simulink model "modelo_f"  (R2024b)
settings: Solver=ode15s  StartTime=0.0  StopTime=inf  FixedStep=T_s  RelTol=1e-3
InitFcn:
  | clc
  | clear
  | close all
  | clear all
  | clear mex
  | parametros
  | gain_CL
  | calculo_observador_carro
  | calculo_observador_izaje
values from neighbouring files (symbols this model uses):
  b_cx = 1e6    (= 1000000)    [parametros.m]
  b_cy = 1e7    (= 10000000)    [parametros.m]
  b_hb = 1e8    (= 100000000)    [parametros.m]
  b_hd = 8    [parametros.m]
  b_hm = 18    [parametros.m]
  b_t = 90    [parametros.m]
  b_tb = 5e6    (= 5000000)    [parametros.m]
  b_td = 1.8    [parametros.m]
  b_tm = 6    [parametros.m]
  b_tw = 3e3    (= 3000)    [parametros.m]
  b_wu = 150    [parametros.m]
  container_pillars = container_pillars(randperm(19))    [parametros.m]
  dx_grid_lidar = 0.01    [parametros.m]
  escenario = 1    [parametros.m]
  g = 9.80665    [parametros.m]
  H_c = 2.59    [parametros.m]
  H_truck = 1    [parametros.m]
  i_h = 22    [parametros.m]
  i_t = 30    [parametros.m]
  J_hd_hEb = 3800    [parametros.m]
  J_hm_hb = 30    [parametros.m]
  J_td = 1200    [parametros.m]
  J_tm_tb = 7    [parametros.m]
  K_cy = 1.8e9    (= 1800000000)    [parametros.m]
  K_tw = 4.8e5    (= 480000)    [parametros.m]
  k_wu = 2.36e8    (= 236000000)    [parametros.m]
  l_h0 = (Y_t0-y_l0)    (= 38)    [parametros.m]
  l_h_max = Y_t0-y_h_min    (= 65)    [parametros.m]
  l_h_maxE = l_h_max+0.5    (= 65.5)    [parametros.m]
  l_h_min = Y_t0-y_h_max    (= 5)    [parametros.m]
  l_h_minE = l_h_min-0.5    (= 4.5)    [parametros.m]
  Lt = place(At', Ct', polos_deseados)'    [calculo_observador_carro.m]
  M_cmax = 50000    [parametros.m]
  M_cmin = 2000    [parametros.m]
  M_s = 15000    [parametros.m]
  M_t = 30000    [parametros.m]
  r_hd = 0.75    [parametros.m]
  r_td = 0.50    (= 0.5)    [parametros.m]
  T_hbMax = 5e4    (= 50000)    [parametros.m]
  T_hEbMax = 1.1e6    (= 1100000)    [parametros.m]
  T_hmMax = 2e4    (= 20000)    [parametros.m]
  T_s = 0.001    [parametros.m]
  T_s0 = 0.001    [parametros.m]
  T_s1 = 0.020    (= 0.02)    [parametros.m]
  T_s2 = 0.020    (= 0.02)    [parametros.m]
  T_tbMax = 5e3    (= 5000)    [parametros.m]
  T_tmMax = 4e3    (= 4000)    [parametros.m]
  tau_tm = 1e-3    (= 0.001)    [parametros.m]
  theta_hm0 = -l_h0*i_h*2/r_hd    (= -2229.33333333)    [parametros.m]
  theta_tm0 = (x_t0)*i_t/r_td    (= -900)    [parametros.m]
  trucks0 = [0, 0, 0, 0, 0]    [parametros.m]
  v_h_max_load = 1.5    [parametros.m]
  v_h_max_noload = 3    [parametros.m]
  v_lx0 = 0    [parametros.m]
  v_ly0 = 0    [parametros.m]
  v_t0 = 0    [parametros.m]
  v_t_max = 4    [parametros.m]
  W_c = ctrb(A, B_c(:,1))    [CyO_carro.m]    (also in CyO_izaje.m; parametros.m = 2.44)
  w_hm0 = 0    [parametros.m]
  w_hm_min_BRK = 0.005    [parametros.m]
  w_hm_rated = v_h_max_load*2*i_h/r_hd    (= 88)    [parametros.m]
  w_tm0 = (v_t0)*i_t/r_td    (= 0)    [parametros.m]
  w_tm_min_BRK = 0.005    [parametros.m]
  x_c0_left = -35    [parametros.m]
  x_c0_right = 55    [parametros.m]
  x_containers_left_lim = 1.5    [parametros.m]
  x_containers_right_lim = 48.5    [parametros.m]
  x_l0 = x_t0    (= -15)    [parametros.m]
  x_lidar_offset = 3.0    (= 3)    [parametros.m]
  x_t0 = -15    [parametros.m]
  x_t_max = 50    [parametros.m]
  x_t_maxE = x_t_max+0.5    (= 50.5)    [parametros.m]
  x_t_min = -30    [parametros.m]
  x_t_minE = x_t_min-0.5    (= -30.5)    [parametros.m]
  y_h_min = -20    [parametros.m]
  y_l0 = 7    [parametros.m]
  Y_sb = 5.0    (= 5)    [parametros.m]
  Y_t0 = 45    [parametros.m]
undefined symbols (not defined in the file or in its folder): Lh, parametros
libraries: dspnetwork x2, dspsigops x1, simulink x1
(part 4 of 4)

== stateflow chart modelo_f/Chart ==
  state Nivel_1
    state Heartbeat_Generator [parallel]
      settings: executionOrder=1
      state Heartbeat_High
        entry:
        heartbeat = true;
      state Heartbeat_Low
        entry:
        heartbeat = false;
      (default) -> Heartbeat_High
      Heartbeat_Low -> Heartbeat_High : after(200, msec)
      Heartbeat_High -> Heartbeat_Low : after(200, msec)
    state Supervisory_Control [parallel]
      settings: executionOrder=2
      state OFF
        entry:
        BRK_h = false;
        BRK_t = false;
        TLK = false;
        v_t_ref = 0.0;
        dl_h_ref = 0.0;
        sway_ctr_enable = false;
        FC_t_min_alarm = false;
        FC_t_max_alarm = false;
        FC_h_min_alarm = false;
        FC_h_max_alarm = false;
        operation_mode = true;
        sway_ctr_gain = 1;
        container_pillars =zeros(1,19);
        m_est_vec = zeros(1, 500);
        m_est = 15000;
        trolley_moving = true;
        trolley_stopped = false;
        trolley_stopped_complete = false;
        hoist_moving = true;
        hoist_stopped = false;
        x_t_obj = x_t_est;
        x_t_ref = x_t_obj;
        l_h_obj = l_h_sensor;
        l_h_ref = l_h_obj;
        state_SISTEMA_ON = false;
        exit:
        state_SISTEMA_ON = true;
        BRK_t_close = false;
        BRK_h_close = false;
        container_pillars_denied = zeros(1, 19);
      state ON
        state BRK_Logic [parallel]
          settings: executionOrder=1
          state BRK_t_Logic [parallel]
            settings: executionOrder=1
            state BRK_t_Closed
              entry:
              BRK_t = false;
            state BRK_t_Opened
              entry:
              BRK_t = true;
            (default) -> BRK_t_Closed
            BRK_t_Opened -> BRK_t_Closed : [(abs(w_tm_estimada) > w_tm_min_BRK) && BRK_t_close]
            BRK_t_Closed -> BRK_t_Opened : [~BRK_t_close]
          state BRK_h_Logic [parallel]
            settings: executionOrder=2
            state BRK_h_Closed
              entry:
              BRK_h = false;
            state BRK_h_Opened
              entry:
              BRK_h = true;
            (default) -> BRK_h_Closed
            BRK_h_Opened -> BRK_h_Closed : [(abs(w_hm_estimada) > w_hm_min_BRK) && BRK_h_close]
            BRK_h_Closed -> BRK_h_Opened : [~BRK_h_close]
        state TLK_Logic [parallel]
          settings: executionOrder=2
          state Init
          state TLK_Opened
            entry:
            TLK = false;
          state TLK_Closed
            entry:
            TLK = true;
          (default) -> Nivel_1.Supervisory_Control.ON.TLK_Logic.Init
          Nivel_1.Supervisory_Control.ON.TLK_Logic.Init -> TLK_Closed [order 1] : [TLK]
          Nivel_1.Supervisory_Control.ON.TLK_Logic.Init -> TLK_Opened [order 2] : [~TLK]
          TLK_Opened -> TLK_Closed : [cmd_TLK && abs(F_hw_sensor) <= 0]
          TLK_Closed -> TLK_Opened : [~cmd_TLK && abs(F_hw_sensor) <= 0]
        state Sway_Control_Mode [parallel]
          settings: executionOrder=3
          state Sway_Control_ON
            entry:
            sway_ctr_enable = true;
          state Sway_Control_OFF
            entry:
            sway_ctr_enable = false;
          (default) -> Sway_Control_ON
          Sway_Control_ON -> Sway_Control_OFF : [~cmd_sway_ctr || l_h_sensor < 10]
          Sway_Control_OFF -> Sway_Control_ON : [cmd_sway_ctr && l_h_sensor > 11]
        state Limit_Switch [parallel]
          during:
          settings: executionOrder=4
          state Trolley_Min_Logic [parallel]
            settings: executionOrder=1
            state FC_t_Min_High
              entry:
              FC_t_min_alarm = true;
            state FC_t_Min_Low
              entry:
              FC_t_min_alarm = false;
            (default) -> FC_t_Min_Low
            FC_t_Min_Low -> FC_t_Min_High : [FC_carro_min]
            FC_t_Min_High -> FC_t_Min_Low : [~FC_carro_min]
          state Trolley_Max_Logic [parallel]
            settings: executionOrder=2
            state FC_t_Max_High
              entry:
              FC_t_max_alarm = true;
            state FC_t_Max_Low
              entry:
              FC_t_max_alarm = false;
            (default) -> FC_t_Max_Low
            FC_t_Max_Low -> FC_t_Max_High : [FC_carro_max]
            FC_t_Max_High -> FC_t_Max_Low : [~FC_carro_max]
          state Hoist_Min_Logic [parallel]
            settings: executionOrder=3
            state FC_h_Min_High
              entry:
              FC_h_min_alarm = true;
            state FC_h_Min_Low
              entry:
              FC_h_min_alarm = false;
            (default) -> FC_h_Min_Low
            FC_h_Min_Low -> FC_h_Min_High : [FC_izaje_min]
            FC_h_Min_High -> FC_h_Min_Low : [~FC_izaje_min]
          state Hoist_Max_Logic [parallel]
            settings: executionOrder=4
            state FC_h_Max_Low
              entry:
              FC_h_max_alarm = false;
            state FC_h_Max_High
              entry:
              FC_h_max_alarm = true;
            (default) -> FC_h_Max_Low
            FC_h_Max_Low -> FC_h_Max_High : [FC_izaje_max]
            FC_h_Max_High -> FC_h_Max_Low : [~FC_izaje_max]
        state Lidar_Map [parallel]
          entry:
          land_end_element = floor((0 - x_c0_left)/dx_grid_lidar) + 1;
          land_end_element = max(1, min(lidar_grid_size, land_end_element));
          lidar_map(land_end_element:end) = y_h_min;
          cc = 0;
          during:
          x_lidar = x_t_est + x_lidar_offset;
          grid_element = max(1, min(lidar_grid_size, floor((x_lidar-x_c0_left)/dx_grid_lidar) + 1));
          lidar_map(grid_element) = y_c0_lidar;
          window_idx = round((v_t_max * T_s2) / dx_grid_lidar);
          n_pilares = 19;
          espaciado = (x_containers_right_lim - x_containers_left_lim) / (n_pilares - 1);
          l_h_safe = 45 - max(lidar_map) - 1.5 * H_c;
          for i = 1:n_pilares
          x_lidar_pillar = x_containers_left_lim + (i-1)*espaciado;
          grid_element_pillar = max(1, min(lidar_grid_size, floor((x_lidar_pillar - x_c0_left)/dx_grid_lidar) + 1));
          window_start = max(1, grid_element_pillar - window_idx);
          window_end   = min(lidar_grid_size, grid_element_pillar + window_idx);
          pillar_height = max(lidar_map(window_start:window_end));
          containers_height = pillar_height - y_h_min;
          container_pillars(i) = max(0, ceil(containers_height / H_c - 1e-6));
          end
          settings: executionOrder=5
        state BRK_Commander [parallel]
          settings: executionOrder=11
          state BRK_t_Activation_Logic [parallel]
            settings: executionOrder=1
            state BRK_t_Free
              entry:
              BRK_t_close = false;
            state BRK_t_Demand
              entry:
              BRK_t_close = true;
            (default) -> BRK_t_Free
            BRK_t_Free -> BRK_t_Demand : [abs(x_t_est - x_t_ref) < 0.01 && abs(v_t_est) < 0.01]
            BRK_t_Demand -> BRK_t_Free : [abs(x_t_est - x_t_ref) > 0.03]
          state BRK_h_Activation_logic [parallel]
            settings: executionOrder=2
            state BRK_h_Free
              entry:
              BRK_h_close = false;
            state BRK_h_Demand
              entry:
              BRK_h_close = true;
            (default) -> BRK_h_Free
            BRK_h_Demand -> BRK_h_Free : [abs(l_h_sensor - l_h_ref) > 0.05]
            BRK_h_Free -> BRK_h_Demand : [abs(l_h_sensor - l_h_ref) < 0.01 && abs(dl_h_est) < 0.01]
        state Any_Alarms [parallel]
          settings: executionOrder=12
          state No_Alarms
            entry:
            alarms = false;
          state Alarms
            entry:
            alarms = true;
          (default) -> No_Alarms
          Alarms -> No_Alarms : [~FC_t_min_alarm && ~FC_t_max_alarm && ~FC_h_min_alarm && ~FC_h_max_alarm]
          No_Alarms -> Alarms : [FC_t_min_alarm || FC_t_max_alarm || FC_h_min_alarm || FC_h_max_alarm]
        state Trolley_Movement_Flags [parallel]
          settings: executionOrder=8
          state Trolley_Moving
            entry:
            trolley_moving = true;
            trolley_stopped = false;
            trolley_stopped_complete = false;
          state Trolley_Stopped
            entry:
            trolley_moving = false;
            trolley_stopped = true;
            trolley_stopped_complete = false;
          state Trolley_Stopped_Complete
            entry:
            trolley_moving = false;
            trolley_stopped = true;
            trolley_stopped_complete = true;
          (default) -> Trolley_Moving
          Trolley_Moving -> Trolley_Stopped : [abs(x_t_est-x_t_obj) <= 0.01 && abs(v_t_est) <= 0.01]
          Trolley_Stopped_Complete -> Trolley_Moving [order 2] : [abs(x_t_est-x_t_obj) > 0.15 || abs(v_t_est) > 0.15]
          Trolley_Stopped -> Trolley_Moving [order 1] : [abs(x_t_est-x_t_obj) > 0.1 || abs(v_t_est) > 0.1]
          Trolley_Stopped -> Trolley_Stopped_Complete [order 2] : [abs(w_l_sensor) <= 0.005 && abs(theta_l_sensor) <= 0.005]
          Trolley_Stopped_Complete -> Trolley_Stopped [order 1] : [abs(w_l_sensor) > 0.005 || abs(theta_l_sensor) > 0.005]
        state Hoist_Movement_Flags [parallel]
          settings: executionOrder=9
          state Hoist_Stopped
            entry:
            hoist_moving = false;
            hoist_stopped = true;
          state Hoist_Moving
            entry:
            hoist_moving = true;
            hoist_stopped = false;
          (default) -> Hoist_Moving
          Hoist_Stopped -> Hoist_Moving : [abs(l_h_sensor-l_h_obj) > 0.1 || abs(dl_h_est) > 0.1]
          Hoist_Moving -> Hoist_Stopped : [abs(l_h_sensor-l_h_obj) <= 0.05 && abs(dl_h_est) <= 0.05]
        state Mode [parallel]
          settings: executionOrder=6
          state Automatic
            during:
          state Manual
            entry:
            v_t_ref_prev = v_t_ref;
            dl_h_ref_prev = dl_h_ref;
            x_t_ref = x_t_est;
            l_h_ref = l_h_sensor;
            during:
            v_t_ref_a = rate_limiter(JS_trolley_cmd*0.15, v_t_ref_prev, 0, T_s1, m_est);
            dl_h_ref_a = rate_limiter(JS_hoist_cmd*0.15, dl_h_ref_prev, 1, T_s1, m_est);
            if FC_t_min_alarm
            v_t_ref = max([0, v_t_ref_a]);
            elseif FC_t_max_alarm
            v_t_ref = min([0, v_t_ref_a]);
            else
            v_t_ref = v_t_ref_a;
            end
            if FC_h_min_alarm
            dl_h_ref = max([0, dl_h_ref_a]);
            elseif FC_h_max_alarm
            dl_h_ref = min([0, dl_h_ref_a]);
            elseif overload
            dl_h_ref = max([0, dl_h_ref_a]);
            else
            dl_h_ref = dl_h_ref_a;
            end
            x_t_ref = x_t_ref + T_s1 * (v_t_ref + v_t_ref_prev)/2;
            l_h_ref = l_h_ref + T_s1 * (dl_h_ref + dl_h_ref_prev)/2;
            v_t_ref_prev = v_t_ref;
            dl_h_ref_prev = dl_h_ref;
          (default) -> Automatic
          Manual -> Automatic : [operation_mode]
          Automatic -> Manual : [~operation_mode]
        state Trajectory_Planner [parallel]
          settings: executionOrder=7
          state Line_Scan_Rise
            entry:
            l_h_obj = l_h_safe;
            [l_h_ref, dl_h_ref, ~, l_h_pr] = generador_trayectoria_izaje(t, l_h_sensor, v_t_est, l_h_obj, m_est, 1);
            during:
            [l_h_ref, dl_h_ref, ~, l_h_pr] = generador_trayectoria_izaje(t, l_h_sensor, v_t_est, l_h_obj, m_est, 0);
          state Scenario_Selector
            entry:
            sway_ctr_gain = 1;
          state Waiting
            entry:
            v_t_ref  = 0;
            dl_h_ref = 0;
          state Line_Scan_Move
            entry:
            x_t_obj = 49.5;
            [x_t_ref, v_t_ref, ~, x_t_pr] = generador_trayectoria(t, x_t_est, x_t_obj, v_t_est, 1);
            during:
            [x_t_ref, v_t_ref, ~, x_t_pr] = generador_trayectoria(t, x_t_est, x_t_obj, v_t_est, 0);
            [l_h_ref, dl_h_ref, ~, l_h_pr] = generador_trayectoria_izaje(t, l_h_sensor, v_t_est, l_h_obj, m_est, 0);
          state Pickup_And_Place_Loop
            exit:
            loop_initialized = true;
            state Init
            state Scenario_Selector
            state Truck_Pickup_Raise
              entry:
              operation_mode = true;
              l_h_obj = l_h_safe;
              [l_h_ref, dl_h_ref, ~, l_h_pr] = generador_trayectoria_izaje(t, l_h_sensor, v_t_est, l_h_obj, m_est, 1);
              during:
              [l_h_ref, dl_h_ref, ~, l_h_pr] = generador_trayectoria_izaje(t, l_h_sensor, v_t_est, l_h_obj, m_est, 0);
              [x_t_ref, v_t_ref, ~, x_t_pr] = generador_trayectoria(t, x_t_est, x_t_obj, v_t_est, 0);
            state Truck_Placement_Manual
              entry:
              operation_mode = false;
              exit:
              m_est = 15000;
            state Truck_Placement_Descend
              entry:
              operation_mode = true;
              l_h_obj = 45 - truck_pickup_height - pickup_safety_margin
              [l_h_ref, dl_h_ref, ~, l_h_pr] = generador_trayectoria_izaje(t, l_h_sensor, v_t_est, l_h_obj, m_est, 1);
              during:
              [l_h_ref, dl_h_ref, ~, l_h_pr] = generador_trayectoria_izaje(t, l_h_sensor, v_t_est, l_h_obj, m_est, 0);
              [x_t_ref, v_t_ref, ~, x_t_pr] = generador_trayectoria(t, x_t_est, x_t_obj, v_t_est, 0);
            state Truck_Pickup_Move
              entry:
              operation_mode = true;
              for i = 1:5
              if trucks_state(i) == 1
              if trucks_has_load(i) == 1
              x_t_obj = -25 + (i-1)*5;
              end
              end
              end
              x_t_obj
              [x_t_ref, v_t_ref, ~, x_t_pr] = generador_trayectoria(t, x_t_est, x_t_obj, v_t_est, 1);
              during:
              [x_t_ref, v_t_ref, ~, x_t_pr] = generador_trayectoria(t, x_t_est, x_t_obj, v_t_est, 0);
              [l_h_ref, dl_h_ref, ~, l_h_pr] = generador_trayectoria_izaje(t, l_h_sensor, v_t_est, l_h_obj, m_est, 0);
            state Truck_Placement_Move
              entry:
              operation_mode = true;
              for i = 1:5
              if trucks_state(i) == 1
              if trucks_has_load(i) == 0
              x_t_obj = -25 + (i-1)*5;
              end
              end
              end
              x_t_obj
              [x_t_ref, v_t_ref, ~, x_t_pr] = generador_trayectoria(t, x_t_est, x_t_obj, v_t_est, 1);
              during:
              [x_t_ref, v_t_ref, ~, x_t_pr] = generador_trayectoria(t, x_t_est, x_t_obj, v_t_est, 0);
              [l_h_ref, dl_h_ref, ~, l_h_pr] = generador_trayectoria_izaje(t, l_h_sensor, v_t_est, l_h_obj, m_est, 0);
            state Truck_Pickup_Descend
              entry:
              operation_mode = true;
              l_h_obj = 45 - truck_pickup_height - pickup_safety_margin
              [l_h_ref, dl_h_ref, ~, l_h_pr] = generador_trayectoria_izaje(t, l_h_sensor, v_t_est, l_h_obj, m_est, 1);
              during:
              [l_h_ref, dl_h_ref, ~, l_h_pr] = generador_trayectoria_izaje(t, l_h_sensor, v_t_est, l_h_obj, m_est, 0);
              [x_t_ref, v_t_ref, ~, x_t_pr] = generador_trayectoria(t, x_t_est, x_t_obj, v_t_est, 0);
            state Truck_Placement_Raise
              entry:
              operation_mode = true;
              l_h_obj = l_h_safe;
              [l_h_ref, dl_h_ref, ~, l_h_pr] = generador_trayectoria_izaje(t, l_h_sensor, v_t_est, l_h_obj, m_est, 1);
              during:
              [l_h_ref, dl_h_ref, ~, l_h_pr] = generador_trayectoria_izaje(t, l_h_sensor, v_t_est, l_h_obj, m_est, 0);
              [x_t_ref, v_t_ref, ~, x_t_pr] = generador_trayectoria(t, x_t_est, x_t_obj, v_t_est, 0);
            state Truck_Pickup_Manual
              entry:
              operation_mode = false;
              m_est_vec_pos = 1;
              m_est_vec(:) = 0;
              during:
              if F_hw_sensor > 8000*g && m_est_vec_pos <= length(m_est_vec(1,:))
              m_est_vec(1, m_est_vec_pos) = 2*F_hw_sensor/g;
              m_est_vec_pos = m_est_vec_pos + 1;
              end
              exit:
              m_est = estimar_masa(m_est_vec);
            state Overload_Check
            state Ship_Pickup_Manual
              entry:
              operation_mode = false;
              m_est_vec_pos = 1;
              m_est_vec(:) = 0;
              during:
              if F_hw_sensor > 8000*g && m_est_vec_pos <= length(m_est_vec(1,:))
              m_est_vec(1, m_est_vec_pos) = 2*F_hw_sensor/g;
              m_est_vec_pos = m_est_vec_pos + 1;
              end
              exit:
              m_est = estimar_masa(m_est_vec);
            state Ship_Placement_Raise
              entry:
              operation_mode = true;
              l_h_obj = l_h_safe;
              [l_h_ref, dl_h_ref, ~, l_h_pr] = generador_trayectoria_izaje(t, l_h_sensor, v_t_est, l_h_obj, m_est, 1);
              during:
              [l_h_ref, dl_h_ref, ~, l_h_pr] = generador_trayectoria_izaje(t, l_h_sensor, v_t_est, l_h_obj, m_est, 0);
              [x_t_ref, v_t_ref, ~, x_t_pr] = generador_trayectoria(t, x_t_est, x_t_obj, v_t_est, 0);
            state Ship_Pickup_Descend
              entry:
              operation_mode = true;
              lidar_map
              l_h_obj = xpos2ypos(lidar_map, x_t_obj) - placement_safety_margin
              [l_h_ref, dl_h_ref, ~, l_h_pr] = generador_trayectoria_izaje(t, l_h_sensor, v_t_est, l_h_obj, m_est, 1);
              during:
              [l_h_ref, dl_h_ref, ~, l_h_pr] = generador_trayectoria_izaje(t, l_h_sensor, v_t_est, l_h_obj, m_est, 0);
              [x_t_ref, v_t_ref,  ~, x_t_pr] = generador_trayectoria(t, x_t_est, x_t_obj, v_t_est, 0);
            state Ship_Placement_Move
              entry:
              operation_mode = true;
              min_containers = 999;
              idx_obj = 1;
              for i = 1:19
              if container_pillars(i) < min_containers
              min_containers = container_pillars(i);
              idx_obj = i;
              end
              end
              espaciado = (x_containers_right_lim - x_containers_left_lim) / (19 - 1);
              x_t_obj = x_containers_left_lim + (idx_obj - 1) * espaciado;
              x_t_obj
              [x_t_ref, v_t_ref, ~, x_t_pr] = generador_trayectoria(t, x_t_est, x_t_obj, v_t_est,1 );
              during:
              [x_t_ref, v_t_ref,  ~, x_t_pr] = generador_trayectoria(t, x_t_est, x_t_obj, v_t_est, 0);
              [l_h_ref, dl_h_ref, ~, l_h_pr] = generador_trayectoria_izaje(t, l_h_sensor, v_t_est, l_h_obj, m_est, 0);
            state Overload_Wait_For_Deposit
            state Ship_Pickup_Move
              entry:
              operation_mode = true;
              max_containers = 0;
              idx_obj = 1;
              for i = 1:19
              if container_pillars(i) > max_containers
              if container_pillars_denied(i) == 0
              max_containers = container_pillars(i);
              idx_obj = i;
              end
              end
              end
              espaciado = (x_containers_right_lim - x_containers_left_lim) / (19 - 1);
              x_t_obj = x_containers_left_lim + (idx_obj - 1) * espaciado;
              x_t_obj
              [x_t_ref, v_t_ref, ~, x_t_pr] = generador_trayectoria(t, x_t_est, x_t_obj, v_t_est,1 );
              during:
              [x_t_ref, v_t_ref,  ~, x_t_pr] = generador_trayectoria(t, x_t_est, x_t_obj, v_t_est, 0);
              [l_h_ref, dl_h_ref, ~, l_h_pr] = generador_trayectoria_izaje(t, l_h_sensor, v_t_est, l_h_obj, m_est, 0);
            state Overload_Ascend_Manual
              during:
              operation_mode = false;
            state Ship_Palcement_Descend
              entry:
              operation_mode = true;
              l_h_obj = xpos2ypos(lidar_map, x_t_obj) - placement_safety_margin
              [l_h_ref, dl_h_ref, ~, l_h_pr] = generador_trayectoria_izaje(t, l_h_sensor, v_t_est, l_h_obj, m_est, 1);
              during:
              [l_h_ref, dl_h_ref, ~, l_h_pr] = generador_trayectoria_izaje(t, l_h_sensor, v_t_est, l_h_obj, m_est, 0);
              [x_t_ref, v_t_ref,  ~, x_t_pr] = generador_trayectoria(t, x_t_est, x_t_obj, v_t_est, 0);
            state Ship_Placement_Manual
              entry:
              operation_mode = false;
              exit:
              m_est = 15000;
            state Ship_Pickup_Raise
              entry:
              operation_mode = true;
              l_h_obj = l_h_safe;
              [l_h_ref, dl_h_ref, ~, l_h_pr] = generador_trayectoria_izaje(t, l_h_sensor, v_t_est, l_h_obj, m_est, 1);
              during:
              [l_h_ref, dl_h_ref, ~, l_h_pr] = generador_trayectoria_izaje(t, l_h_sensor, v_t_est, l_h_obj, m_est, 0);
              [x_t_ref, v_t_ref, ~, x_t_pr] = generador_trayectoria(t, x_t_est, x_t_obj, v_t_est, 0);
            (default) -> Nivel_1.Supervisory_Control.ON.Trajectory_Planner.Pickup_And_Place_Loop.Init
            Nivel_1.Supervisory_Control.ON.Trajectory_Planner.Pickup_And_Place_Loop.Init -> (history) [order 2] : [loop_initialized]
            Nivel_1.Supervisory_Control.ON.Trajectory_Planner.Pickup_And_Place_Loop.Init -> Nivel_1.Supervisory_Control.ON.Trajectory_Planner.Pickup_And_Place_Loop.Scenario_Selector [order 1] : [~loop_initialized]
            Nivel_1.Supervisory_Control.ON.Trajectory_Planner.Pickup_And_Place_Loop.Scenario_Selector -> Ship_Pickup_Raise [order 2] : [escenario == 2]
            Nivel_1.Supervisory_Control.ON.Trajectory_Planner.Pickup_And_Place_Loop.Scenario_Selector -> Truck_Pickup_Raise [order 1] : [escenario == 1 || escenario == 3]
            Truck_Placement_Manual -> Truck_Pickup_Move [order 2] : [(l_h_sensor <=  l_h_obj-1 && ~TLK) && escenario == 3]
            Truck_Placement_Manual -> Ship_Pickup_Raise [order 1] : [(l_h_sensor <=  l_h_obj-1 && ~TLK) && escenario == 2]
            Ship_Placement_Manual -> Truck_Pickup_Raise [order 1] : [(l_h_sensor <=  l_h_obj-1 && ~TLK) && escenario == 1]
            Truck_Placement_Descend -> Truck_Placement_Manual : [hoist_stopped && trolley_stopped_complete]
            Truck_Pickup_Raise -> Truck_Pickup_Move : [hoist_stopped || l_h_pr > 0.8]
            Truck_Placement_Move -> Truck_Placement_Descend : [trolley_stopped]
            Truck_Pickup_Move -> Truck_Pickup_Descend : [trolley_stopped_complete || x_t_pr > 0.95]
            Truck_Placement_Raise -> Truck_Placement_Move : [hoist_stopped || l_h_pr > 0.8]
            Truck_Pickup_Descend -> Truck_Pickup_Manual : [hoist_stopped && trolley_stopped_complete]
            Overload_Check -> Truck_Placement_Raise [order 1] : [after(1000,msec) && ~overload]
            Overload_Check -> Overload_Wait_For_Deposit [order 2] : [overload]
            Ship_Pickup_Manual -> Overload_Check : [l_h_sensor <=  l_h_obj-1 && TLK]
            Truck_Pickup_Manual -> Ship_Placement_Raise : [l_h_sensor <= l_h_obj-1 && TLK]
            Ship_Pickup_Descend -> Ship_Pickup_Manual : [hoist_stopped]
            Ship_Placement_Raise -> Ship_Placement_Move : [hoist_stopped || l_h_pr > 0.8]
            Ship_Pickup_Move -> Ship_Pickup_Descend : [trolley_stopped_complete]
            Overload_Wait_For_Deposit -> Overload_Ascend_Manual : [~TLK]{m_est = 15000;}
            Ship_Placement_Move -> Ship_Palcement_Descend : [trolley_stopped_complete]
            Overload_Ascend_Manual -> Ship_Pickup_Raise : [l_h_sensor <= l_h_obj]
            Ship_Pickup_Raise -> Ship_Pickup_Move : [hoist_stopped || l_h_pr > 0.8]
            Ship_Palcement_Descend -> Ship_Placement_Manual : [hoist_stopped]
            Ship_Placement_Manual -> Ship_Pickup_Raise [order 2] : [([l_h_sensor <=  l_h_obj-1 && ~TLK]) && escenario == 3]
          state Line_Scan_Return
            entry:
            x_t_obj = -29.5;
            [x_t_ref, v_t_ref, ~, x_t_pr] = generador_trayectoria(t, x_t_est, x_t_obj, v_t_est, 1);
            during:
            [x_t_ref, v_t_ref, ~, x_t_pr] = generador_trayectoria(t, x_t_est, x_t_obj, v_t_est, 0);
            [l_h_ref, dl_h_ref, ~, l_h_pr] = generador_trayectoria_izaje(t, l_h_sensor, v_t_est, l_h_obj, m_est, 0);
          (default) -> Line_Scan_Rise
          Nivel_1.Supervisory_Control.ON.Trajectory_Planner.Scenario_Selector -> Waiting [order 1] : [escenario == 0]
          Line_Scan_Return -> Nivel_1.Supervisory_Control.ON.Trajectory_Planner.Scenario_Selector : [trolley_stopped && hoist_stopped]
          Waiting -> Nivel_1.Supervisory_Control.ON.Trajectory_Planner.Scenario_Selector : [escenario ~= 0]
          Line_Scan_Rise -> Line_Scan_Move : [hoist_stopped || l_h_pr > 0.8]
          Pickup_And_Place_Loop -> Nivel_1.Supervisory_Control.ON.Trajectory_Planner.Scenario_Selector : [alarms]
          Nivel_1.Supervisory_Control.ON.Trajectory_Planner.Scenario_Selector -> Pickup_And_Place_Loop [order 2] : [escenario ~= 0 && ~alarms]
          Line_Scan_Move -> Line_Scan_Return : [trolley_stopped]
        state Overload [parallel]
          settings: executionOrder=10
          state No_Overload
            entry:
            overload = false;
            operation_mode = true;
          state Overload
            entry:
            overload = true;
            operation_mode = false;
            container_pillars_denied(idx_obj) = 1;
          (default) -> No_Overload
          No_Overload -> Nivel_1.Supervisory_Control.ON.Overload.Overload : [m_est > M_cmax+M_s]
          Nivel_1.Supervisory_Control.ON.Overload.Overload -> No_Overload : [m_est < 16000]
      (default) -> OFF
      OFF -> ON : [P_APN ]
      ON -> OFF : [~P_APN || emgy]
  (default) -> Nivel_1
  data: t function_input; x_actual function_input; x_final function_input; v_actual function_input; x_t_star function_output; v_t_star function_output; a_t_star function_output; NEW_TRAJ function_input; progreso function_output; t function_input; l_actual function_input; v_actual function_input; l_h_obj function_input; masa_total function_input; NEW_TRAJ function_input; l_h_star function_output; dl_h_star function_output; ddl_h_star function_output; progreso function_output; lidar_map function_input; x function_input; l_h function_output; v_in function_input; v_prev function_input; tipo function_input; Ts function_input; v_out function_output; masa_total function_input; m_est_vec function_input; m_est function_output; emgy input; v_t_ref output double size=1 =0; BRK_h output boolean size=1; theta_tm_sensor input; theta_hm_sensor input; theta_l_sensor input; w_l_sensor input; w_tm_estimada input; JS_trolley_cmd input; JS_hoist_cmd input; w_hm_estimada input; y_c0_lidar input; P_APN input; P_E input boolean; dl_h_est input; cmd_sway_ctr input; trucks_state input double size=1,5; trucks_has_load input double size=1,5; l_h_sensor input; FC_izaje_min input; FC_izaje_max input; FC_carro_max input; FC_carro_min input; cmd_TLK input; F_hw_sensor input; w_hm_min_BRK parameter; w_tm_min_BRK parameter; sway_ctr_enable output boolean size=1; dl_h_ref output double size=1; dx_grid local double size=1 =0.5; force_manual_mode local; n_grid local; x_idx local; heartbeat output boolean size=1; l_h_max parameter; x_t_max parameter; x_t_min parameter; l_h_minE parameter; x_t_est input; x_lidar_offset parameter; dx_grid_lidar parameter; x_lidar local; grid_element local; x_elements local; lidar_map local double size=lidar_grid_size; TLK output boolean size=1 =false; v_t_est input; a_t_max constant double size=1 =a_t_max; v_t_max constant double size=1 =v_t_max; T_s constant double size=1 =T_s0; x_distance local double; radicando local double; max_delta_v constant double size=1 =a_t_max*T_s0; v_ref_deseada local double size=1; v_f_proyectada local double size=1; v_t_ref_prev local double size=1 =0; v_target local double; delta_v local double size=1; T_s2 constant double =T_s2; d_frenado local; t_init local double size=1 =1; x_t_obj local; force_sway_ctr local double size=1 =1; sway_ctr_gain output double size=1 =1; escenario constant double =escenario; i local; data local; data1 local; data2 local; data3 local; x_c0_left constant double =x_c0_left; container_pillars local size=1,19; lidar_grid_size constant double =lidar_grid_size; x_lidar_pillar local; grid_element_pillar local; x_height local; y_h_min constant double =y_h_min; H_c constant double =H_c; containers_height local; land_end_element local; window_idx local; window_end local; window_start local; pillar_height local; idx_obj local; min_containers local; l_h_obj local; x_t_ref output double size=1; data4 local; PES_dy constant double size=1 =PES_dy; PES_map local double size=lidar_grid_size; N_win_pes local; PES_dilated local; PES_raw local; p_start local; p_end local; x_pillar_center local; pillar_height_m local; half_width_idx local; grid_center local; N_dx local; N_ramp local; PES_2D_offset local; PES_y_offset local; truck_pickup_height constant double size=1 =truck_pickup_height; trolley_moving local; trolley_stopped_complete local; trolley_stopped local; l_h_ref output double size=1 =l_h0; pickup_safety_margin constant double size=1 =pickup_safety_margin; hoist_moving local; hoist_stopped local; placement_safety_margin constant double size=1 =placement_safety_margin; x_c0_right constant double size=1 =x_c0_right; x_containers_left_lim constant double size=1 =x_containers_left_lim; x_containers_right_lim constant double size=1 =x_containers_right_lim; n_pilares local; espaciado local; data5 local; data6 local; data7 local; data8 local; data9 local; a local; c local; cc local; col local; dc local double size=1; dr local; n_cols constant double size=1 =n_cols; n_rows constant double size=1 =n_rows; occ_grid_safety local; r local; row_top local; rr local; x_pillar local; dy_grid local double size=1 =0.5; y_h_max constant double size=1 =y_h_max; occ_grid local double size=n_rows,n_cols =zeros(n_rows,n_cols); occ_grid_value local; x_grid_actual local; y_grid_actual local; occ_grid_actual local; l_h_safe local double size=1 =13; operation_mode output boolean size=1 =1; dl_h_ref_prev local; K_corr_h local; error_l_h local; T_s1 local double size=1 =T_s1; l_h_pr local; x_t_pr local; BRK_t output boolean size=1; m_est output double size=1 =15000; m_est_vec local; m_est_vec_pos local; g constant double size=1 =g; k local; n_validos local; suma local; l_h_min local double size=1 =l_h_min; max_containers local double size=1 =0; dl_h_ref_a local; v_t_ref_a local; loop_initialized local boolean size=1 =false; state_SISTEMA_ON output boolean size=1 =false; FC_h_max_alarm output boolean size=1 =false; FC_h_min_alarm output boolean size=1 =false; FC_t_max_alarm output boolean size=1 =false; FC_t_min_alarm output boolean size=1 =false; idx_fin_lidar local; medio_ancho_lidar_idx local; idx_ini_lidar local; W_c constant double; write_end local; write_start local; BRK_h_close local; BRK_t_close local; M_cmax local size=1 =M_cmax; overload local; alarms local; M_s constant double size=1 =M_s; container_pillars_denied local double size=1,19
  function [x_t_star, v_t_star, a_t_star, progreso] = generador_trayectoria(t, x_actual, x_final, v_actual, NEW_TRAJ):
    | function [x_t_star, v_t_star, a_t_star, progreso] = generador_trayectoria(t, x_actual, x_final, v_actual, NEW_TRAJ)
    | % ---------------------------------------------------------------------
    | % LIMITES OPERATIVOS (Seccion 3.3) - PERFIL EN "S" (Jerk Limitado)
    | % ---------------------------------------------------------------------
    | v_max_limite = 4.0; % [m/s]
    | a_max_limite = 0.8; % [m/s^2]
    | % ---------------------------------------------------------------------
    | % ESTADO PERSISTENTE: memoriza el perfil entre llamadas
    | % ---------------------------------------------------------------------
    | persistent x_inicial t_inicio t_a t_crucero t_total v_crucero d_a d_crucero dir inicializado
    | % ---------------------------------------------------------------------
    | % INICIALIZACION OBLIGATORIA PARA CODEGEN
    | % ---------------------------------------------------------------------
    | if isempty(inicializado)
    | inicializado = false;
    | x_inicial = x_actual;
    | t_inicio = t;
    | t_a = 0;
    | t_crucero = 0;
    | t_total = 0;
    | v_crucero = 0;
    | d_a = 0;
    | d_crucero = 0;
    | dir = 0;
    | end
    | % ---------------------------------------------------------------------
    | % GENERACION DE NUEVA TRAYECTORIA (solo cuando NEW_TRAJ == 1)
    | % ---------------------------------------------------------------------
    | if NEW_TRAJ == 1
    | x_inicial = x_actual;
    | t_inicio = t;
    | D = abs(x_final - x_inicial);
    | dir = sign(x_final - x_inicial);
    | if D == 0
    | t_a = 0; t_crucero = 0; t_total = 0;
    | v_crucero = 0; d_a = 0; d_crucero = 0;
    | else
    | t_a = (pi * v_max_limite) / (2 * a_max_limite);
    | d_a = (v_max_limite * t_a) / 2;
    | if 2 * d_a >= D
    | v_pico = sqrt((2 * a_max_limite * D) / pi);
    | t_a = (pi * v_pico) / (2 * a_max_limite);
    | t_crucero = 0;
    | v_crucero = v_pico;
    | d_crucero = 0;
    | d_a = D / 2;
    | else
    | v_crucero = v_max_limite;
    | d_crucero = D - 2 * d_a;
    | t_crucero = d_crucero / v_crucero;
    | end
    | t_total = 2 * t_a + t_crucero;
    | end
    | inicializado = true;
    | end
    | % ---------------------------------------------------------------------
    | % EVALUACION DEL PERFIL CONGELADO, en funcion del tiempo real t
    | % ---------------------------------------------------------------------
    | t_eff = t - t_inicio;
    | 
    | % Progreso 0-1 en base al tiempo total de la trayectoria congelada
    | if t_total > 0
    |     progreso = t_eff / t_total;
    | else
    |     progreso = 1;
    | end
    | progreso = max(0, min(1, progreso));
    | 
    | if t_a == 0 && t_crucero == 0
    | x_t_star = x_final;
    | v_t_star = 0;
    | a_t_star = 0;
    | elseif t_eff < t_a
    | a_t_star = a_max_limite * sin(pi * t_eff / t_a) * dir;
    | v_t_star = (a_max_limite * t_a / pi) * (1 - cos(pi * t_eff / t_a)) * dir;
    | x_t_star = x_inicial + ((a_max_limite * t_a / pi) * (t_eff - (t_a / pi) * sin(pi * t_eff / t_a))) * dir;
    | elseif t_eff < (t_a + t_crucero)
    | t_fase2 = t_eff - t_a;
    | a_t_star = 0;
    | v_t_star = v_crucero * dir;
    | x_t_star = x_inicial + d_a * dir + v_crucero * t_fase2 * dir;
    | elseif t_eff < t_total
    | t_fase3 = t_eff - (t_a + t_crucero);
    | a_t_star = -a_max_limite * sin(pi * t_fase3 / t_a) * dir;
    | v_t_star = (v_crucero - (a_max_limite * t_a / pi) * (1 - cos(pi * t_fase3 / t_a))) * dir;
    | x_t_star = x_inicial + (d_a + d_crucero) * dir + (v_crucero * t_fase3 - (a_max_limite * t_a / pi) * (t_fase3 - (t_a / pi) * sin(pi * t_fase3 / t_a))) * dir;
    | else
    | x_t_star = x_final;
    | v_t_star = 0;
    | a_t_star = 0;
    | end
  function [l_h_star, dl_h_star, ddl_h_star, progreso] = generador_trayectoria_izaje(t, l_actual, v_actual, l_h_obj, masa_total, NEW_TRAJ):
    | function [l_h_star, dl_h_star, ddl_h_star, progreso] = generador_trayectoria_izaje(t, l_actual, v_actual, l_h_obj, masa_total, NEW_TRAJ)
    |     % Parámetros físicos
    |     m_l_nom = 65000;             % [kg] Masa suspendida nominal máxima (M_s + M_c_max)
    |     g_local = 9.80665;
    |     v_h_max_noload = 3.0;    % [m/s] Límite absoluto sin carga (spreader vacío)
    |     v_h_max_load   = 1.5;    % [m/s] Límite absoluto con carga nominal máxima
    |     
    |     % P_const se deriva de los límites de arriba para que la hipérbola
    |     % de potencia constante sea siempre consistente con ellos.
    |     P_const = m_l_nom * g_local * v_h_max_load;
    |     
    |     a_max_limite = 0.75*0.35;
    |     
    |     % Variables persistentes (estado interno)
    |     persistent t_inicio inicializado 
    |     persistent l_ini l_fin ta tc td tt
    |     persistent v0 vp da dc dd dir
    |     persistent v_ult_manual % <--- Memoria para blindar la transición
    |     
    |     if isempty(inicializado)
    |         inicializado = false;
    |         t_inicio = t;
    |         l_ini = l_actual; l_fin = l_actual;
    |         ta = 0; tc = 0; td = 0; tt = 0;
    |         v0 = 0; vp = 0; da = 0; dc = 0; dd = 0; dir = 0;
    |         v_ult_manual = 0;
    |     end
    |     
    |     % Si estamos en manual o fuera de transición, guardamos la velocidad que trae
    |     if NEW_TRAJ == 0
    |         v_ult_manual = v_actual;
    |     end
    |     
    |     % -----------------------------------------------------------------
    |     % PLANIFICACIÓN DE LA TRAYECTORIA (NEW_TRAJ == 1)
    |     % -----------------------------------------------------------------
    |     if NEW_TRAJ == 1
    |         t_inicio = t;
    |         
    |         % Velocidad máxima según hipérbola de potencia constante,
    |         % saturada entre los dos límites absolutos (vacío / carga nominal máxima)
    |         v_potencia   = P_const / (masa_total * g_local);
    |         v_max_limite = min(v_h_max_noload, max(v_h_max_load, v_potencia));
    |         
    |         l_ini = l_actual;
    |         l_fin = l_h_obj;
    |         
    |         D   = abs(l_fin - l_ini);
    |         dir = sign(l_fin - l_ini);
    |         
    |         if D < 1e-6
    |             ta = 0; tc = 0; td = 0; tt = 0;
    |             v0 = 0; vp = 0; da = 0; dc = 0; dd = 0; dir = 0;
    |         else
    |             % PROTECCIÓN CONTRA CERO EN TRANSICIÓN:
    |             % Si v_actual llega en 0 pero veníamos con velocidad guardada, usamos la memoria.
    |             v_efectiva = v_actual;
    |             if abs(v_efectiva) < 1e-3 && abs(v_ult_manual) > 1e-3
    |                 v_efectiva = v_ult_manual;
    |             end
    |             
    |             v0 = v_efectiva * dir;
    |             
    |             if v0 > 0
    |                 D_stop_min = (v0^2) / a_max_limite; 
    |             else
    |                 D_stop_min = 0;
    |             end
    |             
    |             umbral_v0_alta = 0.5 * v_max_limite;
    |             umbral_D_cerca = 2.0;
    |             
    |             if D <= D_stop_min && v0 > 0
    |                 vp = v0;
    |                 ta = 0; da = 0;
    |                 tc = 0; dc = 0;
    |                 td = 2 * D / v0; 
    |                 dd = D;
    |             elseif (v0 > umbral_v0_alta && D < umbral_D_cerca && v0 > 0)
    |                 vp = v0;
    |                 ta = 0; da = 0;
    |                 tc = 0; dc = 0;
    |                 td = 2 * D / v0; 
    |                 dd = D;
    |                 tt = td;
    |             else
    |                 vp_req = sqrt((a_max_limite * D + v0^2) / 2); 
    |                 
    |                 if vp_req <= v_max_limite
    |                     vp = vp_req;
    |                     if v0 > vp
    |                         vp = v0;
    |                     end
    |                     ta = 2 * (vp - v0) / a_max_limite;
    |                     da = (v0 + vp) / 2 * ta;
    |                     tc = 0;
    |                     dc = 0;
    |                     td = 2 * vp / a_max_limite;
    |                     dd = (vp / 2) * td;
    |                 else
    |                     vp = v_max_limite;
    |                     if v0 > vp
    |                         vp = v0; 
    |                     end
    |                     ta = 2 * (vp - v0) / a_max_limite;
    |                     da = (v0 + vp) / 2 * ta;
    |                     td = 2 * vp / a_max_limite;
    |                     dd = (vp / 2) * td;
    |                     dc = D - da - dd;
    |                     if dc < 0
    |                         dc = 0;
    |                     end
    |                     tc = dc / vp;
    |                 end
    |             end
    |             tt = ta + tc + td;
    |         end
    |         inicializado = true;
    |     end
    |     
    |     % -----------------------------------------------------------------
    |     % EVALUACIÓN EN TIEMPO REAL
    |     % -----------------------------------------------------------------
    |     t_local = t - t_inicio;
    |     
    |     if tt > 0
    |         progreso = t_local / tt;
    |     else
    |         progreso = 1;
    |     end
    |     progreso = max(0, min(1, progreso));
    |     
    |     if t_local >= tt || tt == 0
    |         l_h_star   = l_fin;
    |         dl_h_star  = 0;
    |         ddl_h_star = 0;
    |     elseif t_local < ta && ta > 0
    |         delta_v = vp - v0;
    |         ddl_h_star = (delta_v / ta) * (1 - cos(2*pi*t_local/ta)) * dir;
    |         dl_h_star  = (v0 + (delta_v / ta) * (t_local - (ta/(2*pi))*sin(2*pi*t_local/ta))) * dir;
    |         l_h_star   = l_ini + (v0*t_local + (delta_v / ta) * ((t_local^2/2) + (ta^2/(4*pi^2))*(cos(2*pi*t_local/ta)-1))) * dir;
    |     elseif t_local < (ta + tc)
    |         t2 = t_local - ta;
    |         ddl_h_star = 0;
    |         dl_h_star  = vp * dir;
    |         l_h_star   = l_ini + (da + vp*t2) * dir;
    |     elseif t_local < tt && td > 0
    |         t3 = t_local - (ta + tc);
    |         ddl_h_star = (-vp / td) * (1 - cos(2*pi*t3/td)) * dir;
    |         dl_h_star  = (vp - (vp / td) * (t3 - (td/(2*pi))*sin(2*pi*t3/td))) * dir;
    |         l_h_star   = l_ini + (da + dc + vp*t3 - (vp / td) * ((t3^2/2) + (td^2/(4*pi^2))*(cos(2*pi*t3/td)-1))) * dir;
    |     else
    |         l_h_star   = l_fin;
    |         dl_h_star  = 0;
    |         ddl_h_star = 0;
    |     end
    | end
  function l_h = xpos2ypos(lidar_map, x):
    | function l_h = xpos2ypos(lidar_map, x)
    | 
    | persistent dx_grid_lidar_local lidar_grid_size_local x_c0_left_local;
    | 
    | if isempty(dx_grid_lidar_local)
    | 
    |     dx_grid_lidar_local = 0.01;
    |     lidar_grid_size_local = 9001;
    |     x_c0_left_local = -35;
    | end
    | 
    | grid_element_local = max(1, min(lidar_grid_size_local, floor((x-x_c0_left_local)/dx_grid_lidar_local) + 1));
    | l_h = 45 - lidar_map(grid_element_local);
    | 
    | end
  function v_out = rate_limiter(v_in, v_prev, tipo, Ts, masa_total):
    | function v_out = rate_limiter(v_in, v_prev, tipo, Ts, masa_total)
    | % v_in       : velocidad deseada (setpoint) a la entrada
    | % v_prev     : velocidad de salida del paso anterior (estado)
    | % tipo       : 0 = trolley/carro, 1 = hoist
    | % Ts         : paso de tiempo (sample time)
    | % masa_total : masa total izada (solo relevante para tipo == 1)
    | 
    |     a_t_max_local = 0.8*0.9;
    |     a_h_max_local = 0.75*0.9;
    |     P_const       = 956150;
    |     g_local       = 9.80665;
    |     m_min         = 10000;   % masa minima plausible (spreader vacio), evita div/0
    | 
    |     if tipo == 0
    |         a_max = a_t_max_local;
    |     else
    |         a_max = a_h_max_local;
    |         % Limite de velocidad por potencia constante.
    |         % Se aplica ANTES del limitador de pendiente: asi, si m_est sube de
    |         % golpe, la consigna desacelera hacia el nuevo limite respetando
    |         % a_max en lugar de saltar en un paso.
    |         v_max_potencia = P_const / (max(masa_total, m_min) * g_local);
    |         % Solo restringe el sentido de izaje (dl_h > 0 = subir, ajustar
    |         % si tu convencion de signo es la inversa).
    |         v_in = min(v_in, v_max_potencia);
    |     end
    | 
    |     dv_max = a_max * Ts;
    |     dv     = v_in - v_prev;
    |     dv     = max(-dv_max, min(dv_max, dv));
    |     v_out  = v_prev + dv;
    | end
  function m_est = estimar_masa(m_est_vec):
    | function m_est = estimar_masa(m_est_vec)
    |     % ---------------------------------------------------------------------
    |     % ESTIMACION DE MASA CON RECHAZO DE OUTLIERS (2 sigma)
    |     % Ignora las posiciones en cero (no validas) y descarta muestras
    |     % que se alejen mas de 2 desviaciones estandar de la media bruta.
    |     % ---------------------------------------------------------------------
    | 
    |     n_elem = length(m_est_vec(1,:));
    | 
    |     % --- Paso 1: media bruta de las muestras validas (no cero) ---
    |     n_validos = 0;
    |     suma = 0;
    |     for k = 1:n_elem
    |         if m_est_vec(1,k) ~= 0
    |             n_validos = n_validos + 1;
    |             suma = suma + m_est_vec(1,k);
    |         end
    |     end
    | 
    |     if n_validos > 0
    |         media_bruta = suma / n_validos;
    | 
    |         % --- Paso 2: desviacion estandar de las muestras validas ---
    |         suma_sq = 0;
    |         for k = 1:n_elem
    |             if m_est_vec(1,k) ~= 0
    |                 suma_sq = suma_sq + (m_est_vec(1,k) - media_bruta)^2;
    |             end
    |         end
    |         std_dev = sqrt(suma_sq / n_validos);
    | 
    |         % --- Paso 3: promedio final excluyendo outliers (> 2 sigma) ---
    |         suma_final = 0;
    |         n_final = 0;
    |         for k = 1:n_elem
    |             if m_est_vec(1,k) ~= 0 && abs(m_est_vec(1,k) - media_bruta) < 2*std_dev
    |                 suma_final = suma_final + m_est_vec(1,k);
    |                 n_final = n_final + 1;
    |             end
    |         end
    | 
    |         if n_final > 0
    |             m_est = suma_final / n_final;
    |         else
    |             m_est = media_bruta; % fallback si el filtro descarto todo (caso raro)
    |         end
    |     else
    |         m_est = 0;
    |     end
    | end
